simulink model "thruster_block"  (R2024a)
settings: Solver=VariableStepAuto  StartTime=0.0  StopTime=10.0  RelTol=1e-3
settings Model: Creator=klyx  LastModifiedBy=nl
settings RTWCC: GPUComputeCapability=3.5

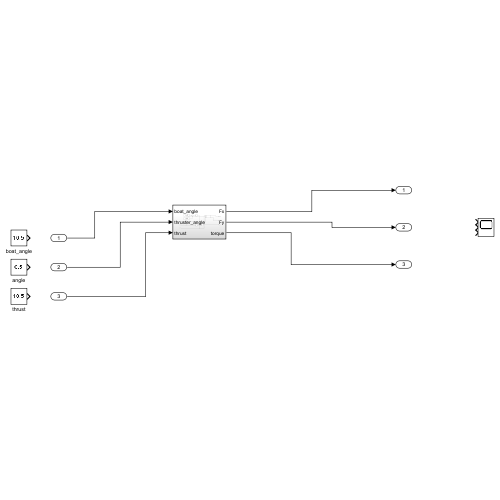
[thumbnail: Simulink's stored preview of the top-level diagram]
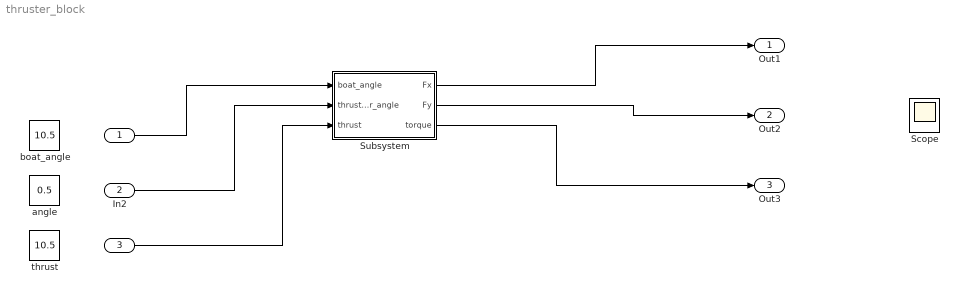
== system thruster_block ==
  " " : Inport
  In2 : Inport  Port=2
  "  " : Inport  Port=3
  Scope : Scope  NumInputPorts=3
  Subsystem : Subsystem
  angle : Constant  Value=0.5
  boat_angle : Constant  Value=10.5
  thrust : Constant  Value=10.5
  Out1 : Outport
  Out2 : Outport  Port=2
  Out3 : Outport  Port=3
  wires:
  " "/1 -> Subsystem/1(boat_angle)
  In2/1 -> Subsystem/2(thruster_angle)
  "  "/1 -> Subsystem/3(thrust)
  Subsystem/1(Fx) -> Out1/1
  Subsystem/2(Fy) -> Out2/1
  Subsystem/3(torque) -> Out3/1

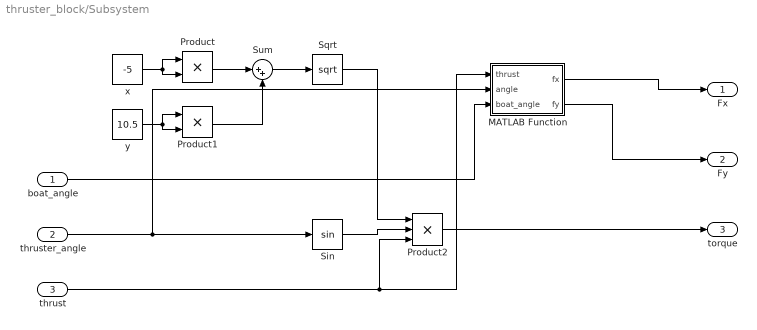
== system thruster_block/Subsystem ==
  boat_angle : Inport
  thruster_angle : Inport  Port=2
  thrust : Inport  Port=3
  MATLAB Function : MATLAB Function  TreatAsAtomicUnit=on
  Product : Product
  Product1 : Product
  Product2 : Product  Inputs=3
  Sin : Trigonometry
  Sqrt : Sqrt
  Sum : Sum  Inputs=|++
  x : Constant  Value=-5
  y : Constant  Value=10.5
  Fx : Outport
  Fy : Outport  Port=2
  torque : Outport  Port=3
  wires:
  Sin/1 -> Product2/2
  Product1/1 -> Sum/2
  y/1 -> Product1/2, Product1/1
  Product/1 -> Sum/1
  thruster_angle/1 -> Sin/1, MATLAB Function/2(angle)
  thrust/1 -> MATLAB Function/1(thrust), Product2/3
  boat_angle/1 -> MATLAB Function/3(boat_angle)
  MATLAB Function/1(fx) -> Fx/1
  MATLAB Function/2(fy) -> Fy/1
  Sum/1 -> Sqrt/1
  Product2/1 -> torque/1
  Sqrt/1 -> Product2/1
  x/1 -> Product/1, Product/2

== matlab function thruster_block/Subsystem/MATLAB Function ==
  data: thrust input; fx output; angle input; boat_angle input; fy output
function [fx,fy] = fcn(thrust, angle, boat_angle)

Rx = [cos(boat_angle) -sin(boat_angle); sin(boat_angle) cos(boat_angle)];
f = [sin(angle); cos(angle)]*thrust;
mf = Rx*f;
fx = mf(1);
fy = mf(2);
